simulink model "lab2_prob2"  (R2024a)
settings: Solver=FixedStepAuto  StartTime=0.0  StopTime=25  FixedStep=0.001  RelTol=1e-3
model workspace (MATLAB code in the model file):
  | k = 40;
  | g = 9.80665;
  | m = 0.25;
  | L = 0.5;
settings Model: Creator=pablo  LastModifiedBy=pablo

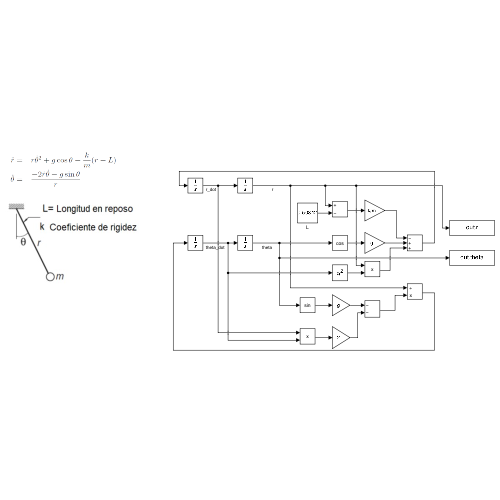
[thumbnail: Simulink's stored preview of the top-level diagram]
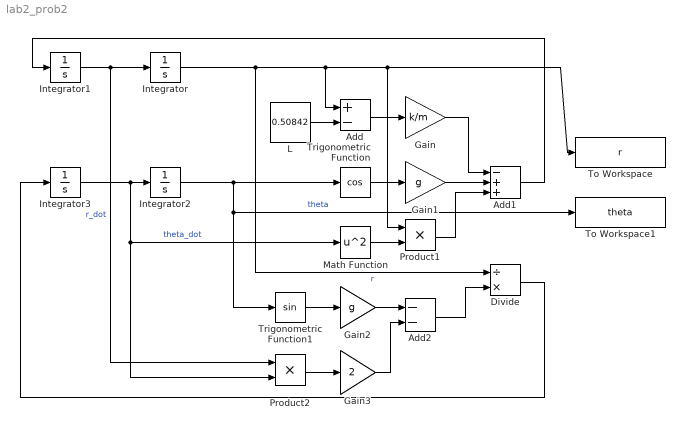
== system lab2_prob2 ==
  Add : Sum  Inputs=+-
  Add1 : Sum  Inputs=-++
  Add2 : Sum  Inputs=--
  Divide : Product  Inputs=/*
  Gain : Gain  Gain=k/m
  Gain1 : Gain  Gain=g
  Gain2 : Gain  Gain=g
  Gain3 : Gain  Gain=2
  Integrator : Integrator  InitialCondition=L
  Integrator1 : Integrator
  Integrator2 : Integrator  InitialCondition=60*pi/180
  Integrator3 : Integrator
  L : Constant  Value=0.50842
  Math Function : Math  Operator=square
  Product1 : Product
  Product2 : Product
  To Workspace : ToWorkspace  VariableName=r  SampleTime=-1
  To Workspace1 : ToWorkspace  VariableName=theta  SampleTime=-1
  Trigonometric Function : Trigonometry  Operator=cos
  Trigonometric Function1 : Trigonometry
  wires:
  Integrator/1 -> To Workspace/1, Product1/1, Add/1, Divide/1  "r"
  Integrator1/1 -> Product2/1, Integrator/1  "r_dot"
  L/1 -> Add/2
  Add/1 -> Gain/1
  Gain/1 -> Add1/1
  Gain1/1 -> Add1/2
  Trigonometric Function/1 -> Gain1/1
  Integrator2/1 -> Trigonometric Function1/1, To Workspace1/1, Trigonometric Function/1  "theta"
  Math Function/1 -> Product1/2
  Product1/1 -> Add1/3
  Add1/1 -> Integrator1/1
  Integrator3/1 -> Product2/2, Math Function/1, Integrator2/1  "theta_dot"
  Trigonometric Function1/1 -> Gain2/1
  Gain2/1 -> Add2/1
  Product2/1 -> Gain3/1
  Gain3/1 -> Add2/2
  Add2/1 -> Divide/2
  Divide/1 -> Integrator3/1
